simulink model "BOOSTWITHPV"  (R2021a)
settings: Solver=VariableStepAuto  StartTime=0.0  StopTime=2  RelTol=1e-3
undefined symbols (not defined in the file): sigbuilder_block
libraries: spsSeriesRLCBranchLib x4, spsDiodeLib x1, spsCurrentMeasurementLib x1, spsMosfetLib x1, spsPVArrayLib x1, spsPWMGeneratorDCDCLib x1, spsVoltageMeasurementLib x1, spspowerguiLib x1
settings Model: Creator=abc  LastModifiedBy=abc

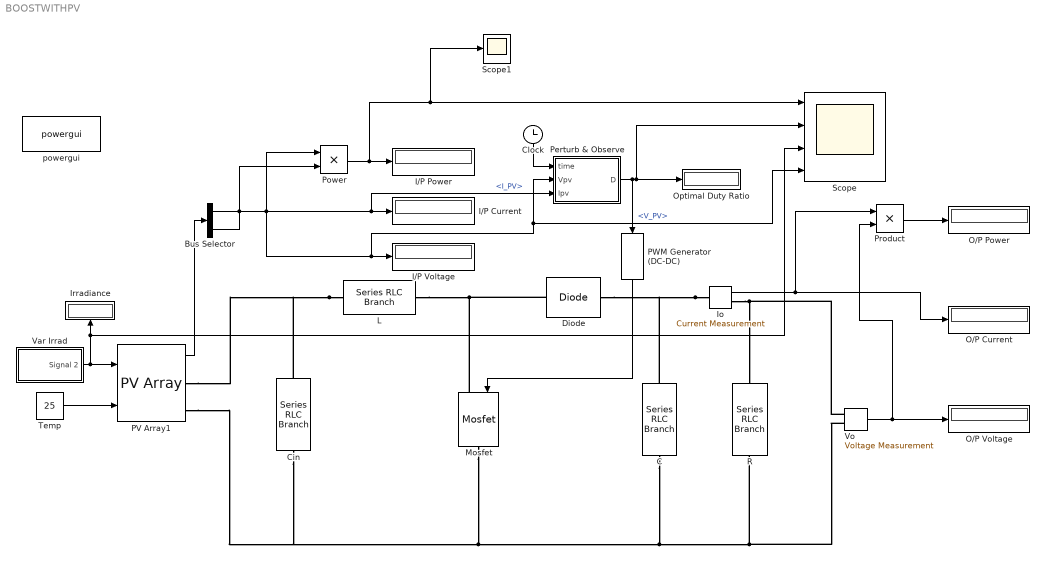
== system BOOSTWITHPV ==
  Bus Selector : BusSelector  OutputSignals=V_PV,I_PV
  C : spsSeriesRLCBranchLib/Series RLC Branch  LConnTagsString=__new0  RConnTagsString=__new0  BranchType=C  Resistance=1  Inductance=1e-3  SetiL0=off  InitialCurrent=0  Capacitance=23.35e-6  Setx0=off  InitialVoltage=0  Measurements=None
  Cin : spsSeriesRLCBranchLib/Series RLC Branch  LConnTagsString=__new0  RConnTagsString=__new0  BranchType=RC  Resistance=0.0001  Inductance=1.875e-4  SetiL0=off  InitialCurrent=0  Capacitance=1000e-6  Setx0=off  InitialVoltage=0  Measurements=None
  Clock : Clock
      settings: Decimation=2
  Diode : spsDiodeLib/Diode  Ron=0.001  Lon=0  Vf=0.8  IC=0  UseSnubber=0  Rs=500  Cs=250e-9  Measurements=off
  I/P Current : Display
  I/P Power : Display
  I/P Voltage : Display
  Io : spsCurrentMeasurementLib/Current Measurement  PhasorSimulation=off  OutputType=Complex  PSBequivalent=0
  Irradiance : Display
  L : spsSeriesRLCBranchLib/Series RLC Branch  LConnTagsString=__new0  RConnTagsString=__new0  BranchType=L  Resistance=1  Inductance=62.928e-3  SetiL0=off  InitialCurrent=0  Capacitance=1e-6  Setx0=off  InitialVoltage=0  Measurements=None
  Mosfet : spsMosfetLib/Mosfet  Ron=0.1  Lon=0  Rd=0.01  Vfd=0  IC=0  Rs=1e5  Cs=inf  Measurements=off
  O/P Current : Display
  O/P Power : Display
  O/P Voltage : Display
  Optimal Duty Ratio : Display
  PV Array1 : spsPVArrayLib/PV Array  Npar=1  Nser=1  PlotType=array @ 25 deg.C & specified irradiances  S_vec="[ 1000  500  100 ]"  Temp_C_vec=[1000 500 100]  ModuleName=User-defined  PlotWhenSelected=off  Pm=10.004  Ncell=60  Voc=21  Isc=0.709  Vm=16.4  Im=0.610  beta_Voc_pc=-0.36099  alpha_Isc_pc=0.102  beta_Voc=-0.075808  alpha_Isc=0.00072318  IL=0.71857  I0=2.5658e-11  nI=0.5693  Rsh=246.0147  Rs=3.3198  RobustModel=off  RobustCellTemperature=313.3991  BAL=on  Tc=1e-6  Tfilter=5e-5
  PWM Generator (DC-DC) : spsPWMGeneratorDCDCLib/PWM Generator (DC-DC)  Fsw=15000  Ts=10e-6
  Perturb & Observe : MATLAB Function  TreatAsAtomicUnit=on
  Power : Product
  Product : Product
  R : spsSeriesRLCBranchLib/Series RLC Branch  LConnTagsString=__new0  RConnTagsString=__new0  BranchType=R  Resistance=300  Inductance=1e-3  SetiL0=off  InitialCurrent=0  Capacitance=1e-6  Setx0=off  InitialVoltage=0  Measurements=None
  Scope : Scope  NumInputPorts=4
  Scope1 : Scope
  Temp : Constant  Value=25
  Var Irrad : Subsystem  Tag=STV Subsys  LoadFcn=sigbuilder_block('load');  StartFcn=sigbuilder_block('start');  StopFcn=sigbuilder_block('stop');  ClipboardFcn=sigbuilder_block('clipboard');  mask(Sigbuilder block){tuvar=[0:10]}
      mask help: Simulink:masks:SigbuilderBlock_MD
      mask init:
      | if ~strcmp(get_param(bdroot(gcbh),'SimulationStatus'),'stopped') tuvar = sigbuilder_block('maskInit'); end
      settings: CopyFcn=sigbuilder_block('copy');  DeleteFcn=sigbuilder_block('delete');  ModelCloseFcn=sigbuilder_block('modelClose');  PreSaveFcn=sigbuilder_block('preSave');  PauseFcn=sigbuilder_block('pause');  ContinueFcn=sigbuilder_block('continue');  NameChangeFcn=sigbuilder_block('namechange');  OpenFcn=sigbuilder_block('open',[381.6 96.6 550.8 400.2 ]);  CloseFcn=sigbuilder_block('close');
      mask Display: plot(0, 0, 100, 100,[2, 2, 32, 32, 2], [68, 8, 8, 68, 68],[32, 2], [38, 38], [32, 19, 2],[53, 60, 44], [32, 17, 17, 2],[16, 16, 31, 31]);txt = getActiveGroup(gcbh);text(2, 100, txt,'verticalAlignment', 'top');
  Vo : spsVoltageMeasurementLib/Voltage Measurement  PhasorSimulation=off  OutputType=Complex  PSBequivalent=0
  powergui : spspowerguiLib/powergui  Priority=1  SimulationMode=Discrete  SampleTime=1e-6  frequency=60  Iterations=50  frequencyindice=0  Pbase=100e6  ErrMax=1e-4  UnitsV=kV  UnitsW=MW  buscounter=0  FunctionMessages=off  echomessages=off  EnableUseOfTLC=off  CurrentSourceSwitches=off  DisableSnubberDevices=off  DisableRonSwitches=off  DisableVfSwitches=off  DisplayEquations=off  AutomaticDiscreteSolvers=off  SolverType=Tustin/Backward Euler (TBE)  Interpol=off  ExternalGateDelay=off  methode=off  Ts=100  x0status=blocks  SPID=on  SwTol=0  HookPort=off  NonlinearTolerance=1e-4  nMaxIteration=100  ContinueOnMaxIteration=off  RestoreLinks=warning  ResistiveCurrentMeasurement=off  Frange=[0:2:500]  Ylog=off  Xlog=on  ShowGrid=off  save=off  variable=ZData  structure=0  ZoomFFT=off  StartTime=0.0  cycles=1  DisplayStyle=1  fundamental=60  FreqAxis=off  MaxFrequency=1000  frequencyindicesteady=1  RmsSteady=1  display=off
  wires:
  Power/1 -> Scope1/1, Scope/1, I/P Power/1
  Bus Selector/1 -> Scope/4, Perturb & Observe/2(Vpv), I/P Voltage/1, Power/1  "<V_PV>"
  PWM Generator (DC-DC)/1 -> Mosfet/1
  Clock/1 -> Perturb & Observe/1(time)
  Vo/1 -> Product/2, O/P Voltage/1
  Io/1 -> O/P Current/1, Product/1
  PV Array1/1 -> Bus Selector/1
  Product/1 -> O/P Power/1
  Perturb & Observe/1(D) -> Optimal Duty Ratio/1, Scope/2, PWM Generator (DC-DC)/1
  Bus Selector/2 -> Power/2, Perturb & Observe/3(Ipv), I/P Current/1  "<I_PV>"
  Temp/1 -> PV Array1/2
  Var Irrad/1(Signal 2) -> PV Array1/1, Scope/3, Irradiance/1
  connections:
  C/RConn1 -- Mosfet/RConn1 -- PV Array1/RConn2 -- Cin/RConn1 -- R/RConn1 -- Vo/LConn2
  Vo/LConn1 -- Io/RConn1 -- R/LConn1
  L/LConn1 -- PV Array1/RConn1 -- Cin/LConn1
  Mosfet/LConn1 -- L/RConn1 -- Diode/LConn1
  Io/LConn1 -- C/LConn1 -- Diode/RConn1

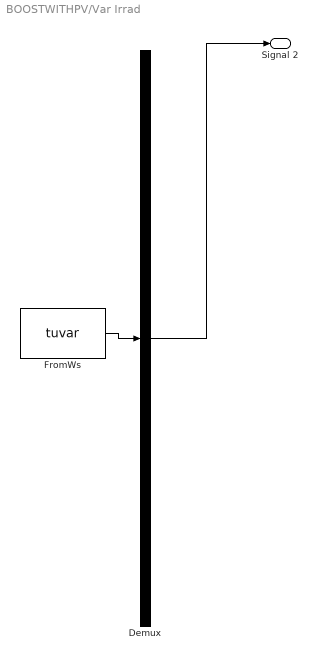
== system BOOSTWITHPV/Var Irrad ==
  Demux : Demux  Tag=STV Demux  Outputs=1
      settings: DisplayOption=none
  FromWs : FromWorkspace  Tag=STV FromWs  VariableName=tuvar
      SigBuilderData=|
      | common.afterFinalStr = 'Extrapolate'
      | common.sampleTime = 0
      | dataSet.timeRange = [0 2]
      | dataSet.name = 'Group 1'
      | sbobj.Groups.Name = 'Group 1'
      | sbobj.Groups.Signals.Name = 'Signal 2'
      | sbobj.Groups.Signals.XData = [0 0.5 0.5 1 1 1.5 1.5 2]
      | sbobj.Groups.Signals.YData = [1000 1000 600 600 800 800 1000 1000]
      | sbobj.Groups.TimeRange = [0 2]
  Signal 2 : Outport  Tag=STV Outport
  wires:
  FromWs/1 -> Demux/1
  Demux/1 -> Signal 2/1

== matlab function BOOSTWITHPV/Perturb & Observe ==
  data: time input; Vpv input; D output; Ipv input
function D = PO(time, Vpv, Ipv)

persistent Dprev Vprev Pprev prevTime

if isempty(prevTime)
    prevTime = 0;
    Dprev = 0.7;
    Vprev = Vpv;
    Pprev = Vpv * Ipv;
end

dT = time - prevTime;
delD = 0.01;
timeStep = 0.01;

if dT >= timeStep && time >= 0.1
    Ppv = Vpv * Ipv;
    dP = Ppv - Pprev;
    dV = Vpv - Vprev;
    if dP ~= 0
        if dP > 0
            if dV > 0
                % left side of MPP
                D = Dprev - delD;
            else
                % right side of MPP
                D = Dprev + delD;
            end
        else
            if dV > 0
                % right side of MPP
                D = Dprev + delD;
            else
                % left side of MPP
                D = Dprev - delD;
            end
        end
    else
        % MPP reached
        D = Dprev;
    end
    % Store current values in the previous variables
    Dprev = D;
    prevTime = time;
    Pprev = Ppv;
    Vprev = Vpv;
else
    % MPPT is not engaged
    D = Dprev;
end

end
